simulink model "LKAS"  (R2018a)
settings: Solver=VariableStepAuto  StartTime=0.0  StopTime=50  RelTol=1e-3
undefined symbols (not defined in the file): gray, Rec, SDTV
libraries: visiongeotforms x4, visionsinks x4, vrlib x4, visionconversions x2, visiontextngfix x2, simulink x1, dspvision x1
settings Model: Creator=Aral_Sarrafi  LastModifiedBy=Aral_Sarrafi

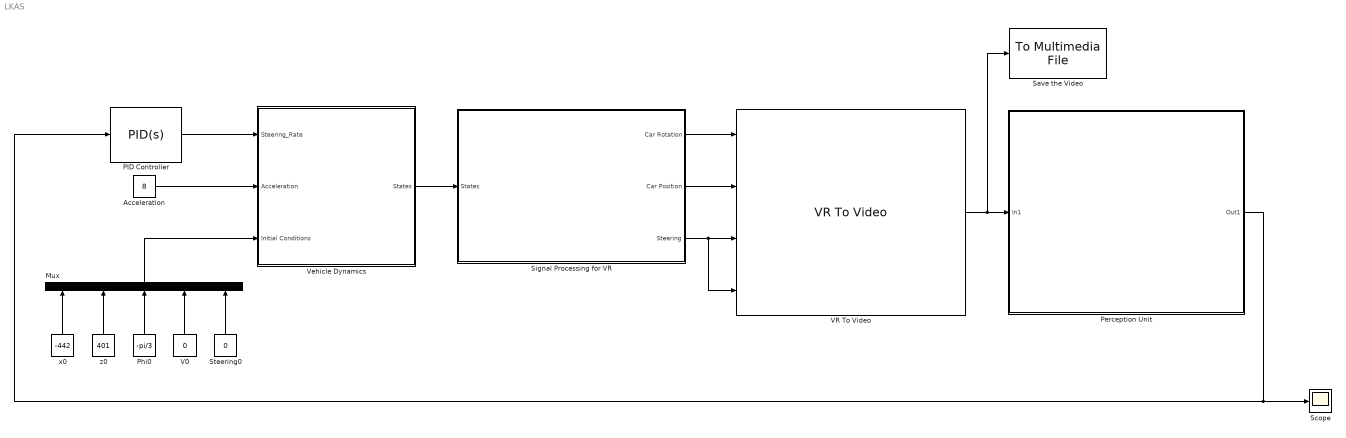
== system LKAS ==
  Acceleration : Constant  Value=8
  Mux : Mux  Inputs=5
  PID Controller : simulink/Continuous/PID Controller  Controller=PID  TimeDomain=Continuous-time  SampleTime=-1  IntegratorMethod=Forward Euler  FilterMethod=Forward Euler  Form=Parallel  UseFilter=on  ControllerParametersSource=internal  P=0.015  I=0.02  D=0.012  N=100  InitialConditionSource=internal  InitialConditionForIntegrator=0  InitialConditionForFilter=0  ExternalReset=none  LimitOutput=on  UpperSaturationLimit=pi/2  LowerSaturationLimit=-pi/2  LinearizeAsGain=off  AntiWindupMode=back-calculation  Kb=1  TrackingMode=off  Kt=1  PParamMin=[]  PParamMax=[]  IParamMin=[]  IParamMax=[]  DParamMin=[]  DParamMax=[]  NParamMin=[]  NParamMax=[]  KbParamMin=[]  KbParamMax=[]  KtParamMin=[]  KtParamMax=[]  POutMin=[]  POutMax=[]  IOutMin=[]  IOutMax=[]  DOutMin=[]  DOutMax=[]  NOutMin=[]  NOutMax=[]  KbOutMin=[]  KbOutMax=[]  KtOutMin=[]  KtOutMax=[]  IntegratorOutMin=[]  IntegratorOutMax=[]  FilterOutMin=[]  FilterOutMax=[]  SumOutMin=[]  SumOutMax=[]  SumI1OutMin=[]  SumI1OutMax=[]  SumI2OutMin=[]  SumI2OutMax=[]  SumI3OutMin=[]  SumI3OutMax=[]  SumDOutMin=[]  SumDOutMax=[]  SaturationOutMin=[]  SaturationOutMax=[]  IntegratorContinuousStateAttributes=''  IntegratorStateMustResolveToSignalObject=off  IntegratorRTWStateStorageClass=Auto  FilterContinuousStateAttributes=''  FilterStateMustResolveToSignalObject=off  FilterRTWStateStorageClass=Auto  DifferentiatorICPrevScaledInput=0  DifferentiatorOutMin=[]  DifferentiatorOutMax=[]  FilterDiffOutCoefMin=[]  FilterDiffOutCoefMax=[]  SumDenOutMin=[]  SumDenOutMax=[]  SumNumOutMin=[]  SumNumOutMax=[]  ReciprocalOutMin=[]  ReciprocalOutMax=[]  DivideOutMin=[]  DivideOutMax=[]  TunerSelectOption=Transfer Function Based (PID Tuner App)
  Perception Unit : Subsystem
      mask Display: image('computer-vision.jpg');
  Phi0 : Constant  Value=-pi/3
  Save the Video : dspvision/To Multimedia File  outputFilename=Final.mp4  streamSelection=Video only  videoCompressor=DV Video Encoder  audioCompressor=None (uncompressed)  imagePorts=One multidimensional signal  fileType=MPEG4  audioDatatype=Determine from input data type  fourcc=RGB  videoQuality=50  mj2000CompFactor=10
      settings: SourceProductName=Computer Vision System Toolbox  SourceProductBaseCode=VP
  Scope : Scope
  Signal Processing for VR : Subsystem
  Steering0 : Constant  Value=0
  V0 : Constant  Value=0
  VR To Video : vrlib/VR To Video  InstantiateOnLoad=on  SampleTime=0.02  ViewEnable=on  RemoteChange=off  RemoteView=off  FieldsWritten=Car.rotation.4.1.1.double#Car.translation.3.1.1.double#Front1.rotation.4.1.1.double#Front2.rotation.4.1.1.double  WorldFileName=Driving_Track.wrl  AutoView=off  VideoDimensions=[750 1200]  AllowVariableSize=off  FigureProperties="{'Position', 'Name', 'Viewpoint', 'CameraBound', 'CameraDirection', 'CameraPosition', 'CameraUpVector', 'ZoomFactor', 'Antialiasing', 'Headlight', 'Lighting', 'NavPanel', 'Sound', 'StatusBar', 'Stereo3D', 'Stereo3DCameraOffset', 'Stereo3DHIT', 'ToolBar', 'Textures', 'Transparency', 'Triad', 'Wireframe', 'NavZones', 'NavMode', 'NavSpeed', 'CaptureFileFormat', 'CaptureFileName', 'Record2DCompressMethod', 'Record2DCompressQuality', 'Record2D', 'Record2DFileName', 'Record2DFPS'; [3.0000000000000000e+01   6.0000000000000000e+01   1.2000000000000000e+03   7.5000000000000000e+02], '', '_untitled_1', 'on', [0.0000000000000000e+00   0.0000000000000000e+00  -1.0000000000000000e+00], [0.0000000000000000e+00   0.0000000000000000e+00   0.0000000000000000e+00], [0.0000000000000000e+00   1.0000000000000000e+00   0.0000000000000000e+00], [1.0000000000000000e+00], 'on', 'on', 'on', 'none', 'on', 'off', 'off', [1.0000000149011612e-01], [0.0000000000000000e+00], 'off', 'on', 'on', 'none', 'off', 'off', 'fly', 'normal', 'tif', '%f_anim_%n.tif', 'auto', [7.5000000000000000e+01], 'off', '***video***', 'auto'}"
      settings: SourceProductName=Simulink 3D Animation  SourceProductBaseCode=VR
  Vehicle Dynamics : Subsystem
  x0 : Constant  Value=-442
  z0 : Constant  Value=401
  wires:
  VR To Video/1 -> Save the Video/1, Perception Unit/1(In1)
  Perception Unit/1(Out1) -> PID Controller/1, Scope/1
  Signal Processing for VR/1(Car Rotation) -> VR To Video/1
  Signal Processing for VR/2(Car Position) -> VR To Video/2
  Signal Processing for VR/3(Steering) -> VR To Video/4, VR To Video/3
  PID Controller/1 -> Vehicle Dynamics/1(Steering_Rate)
  Vehicle Dynamics/1(States) -> Signal Processing for VR/1(States)
  Acceleration/1 -> Vehicle Dynamics/2(Acceleration)
  V0/1 -> Mux/4
  Phi0/1 -> Mux/3
  z0/1 -> Mux/2
  x0/1 -> Mux/1
  Mux/1 -> Vehicle Dynamics/3(Initial Conditions)
  Steering0/1 -> Mux/5

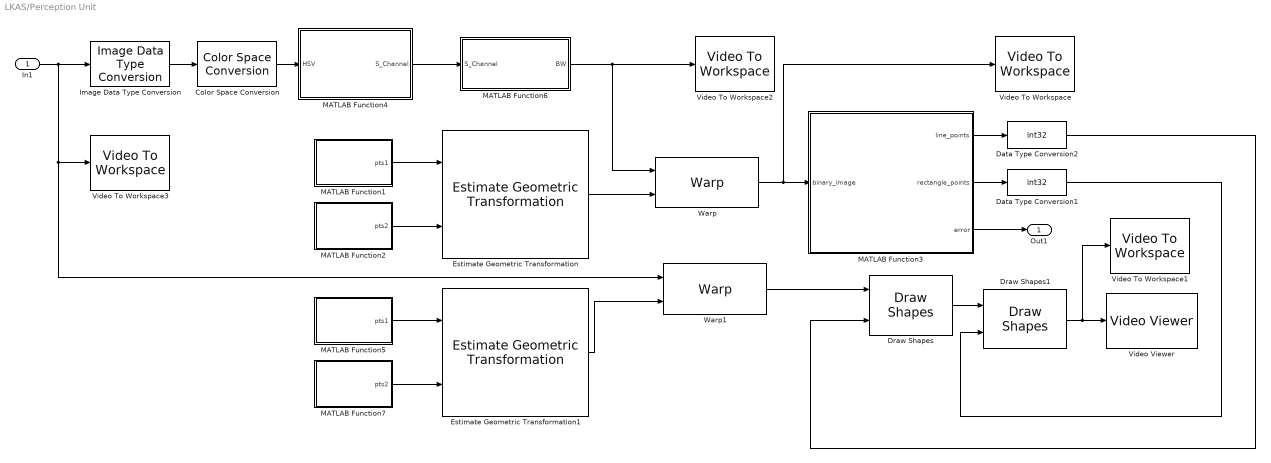
== system LKAS/Perception Unit ==
  In1 : Inport
  Color Space Conversion : visionconversions/Color Space  Conversion  conversion=Obsolete  conversionActive=R'G'B' to HSV  wp_str=D65  rec=Rec. 601 (SDTV)  sys=1125/60/2:1  imagePorts=One multidimensional signal
      settings: SourceProductName=Computer Vision System Toolbox
  Data Type Conversion1 : DataTypeConversion  OutDataTypeStr=int32
  Data Type Conversion2 : DataTypeConversion  OutDataTypeStr=int32
  Draw Shapes : visiontextngfix/Draw Shapes  shape=Lines  fill=off  lineWidth=4  fillClrSource=Specify via dialog  display=User-specified value  intensity=200  color=[255 0 0]  opacity=0.6  viewport=Entire image  antialiasing=off  inType=Obsolete  imagePorts=One multidimensional signal  prodOutputMode=Binary point scaling  prodOutputWordLength=32  prodOutputFracLength=14  memoryMode=Specify word length  memoryWordLength=16  memoryFracLength=14  roundingMode=Floor  overflowMode=off
      settings: SourceProductName=Computer Vision System Toolbox
  Draw Shapes1 : visiontextngfix/Draw Shapes  shape=Rectangles  fill=off  lineWidth=1  fillClrSource=Specify via dialog  display=User-specified value  intensity=200  color=[0 255 0]  opacity=0.6  viewport=Entire image  antialiasing=off  inType=Obsolete  imagePorts=One multidimensional signal  prodOutputMode=Binary point scaling  prodOutputWordLength=32  prodOutputFracLength=14  memoryMode=Specify word length  memoryWordLength=16  memoryFracLength=15  roundingMode=Floor  overflowMode=off
      settings: SourceProductName=Computer Vision System Toolbox
  Estimate Geometric Transformation : visiongeotforms/Estimate Geometric Transformation  tformType=Projective  isRandomSampling=on  algMethod=Random Sample Consensus (RANSAC)  distanceAlg=2.5  distanceGeo=2.5  numMethod=Specified value  sampleNum=500  desiredConfidence=99  maxSampleNum=1000  isStopSampling=off  percentStop=75  isRefineTForm=off  isReleaseMode=on  isOutputInlier=off  outDT4IntInput=Obsolete10a  outDT4IntInputActive=Single  isVarSizeAllowed=on
      settings: SourceProductName=Computer Vision System Toolbox  SourceProductBaseCode=VP
  Estimate Geometric Transformation1 : visiongeotforms/Estimate Geometric Transformation  tformType=Projective  isRandomSampling=on  algMethod=Random Sample Consensus (RANSAC)  distanceAlg=2.5  distanceGeo=2.5  numMethod=Specified value  sampleNum=500  desiredConfidence=99  maxSampleNum=1000  isStopSampling=off  percentStop=75  isRefineTForm=off  isReleaseMode=on  isOutputInlier=off  outDT4IntInput=Obsolete10a  outDT4IntInputActive=Single  isVarSizeAllowed=on
      settings: SourceProductName=Computer Vision System Toolbox  SourceProductBaseCode=VP
  Image Data Type Conversion : visionconversions/Image Data Type Conversion  outDT=double  isSigned=on  wordLen=16  numFracBits=0
      settings: SourceProductName=Computer Vision System Toolbox  SourceProductBaseCode=VP
  MATLAB Function1 : MATLAB Function  TreatAsAtomicUnit=on
  MATLAB Function2 : MATLAB Function  TreatAsAtomicUnit=on
  MATLAB Function3 : MATLAB Function  TreatAsAtomicUnit=on
  MATLAB Function4 : MATLAB Function  TreatAsAtomicUnit=on
  MATLAB Function5 : MATLAB Function  TreatAsAtomicUnit=on
  MATLAB Function6 : MATLAB Function  TreatAsAtomicUnit=on
  MATLAB Function7 : MATLAB Function  TreatAsAtomicUnit=on
  Video To Workspace : visionsinks/Video To Workspace  VariableName=warped  NumInputs=1  DataLimit=251  DecimationFactor=2  LogFi=off  InPortLabels=R|G|B
      settings: SourceProductName=Computer Vision System Toolbox  SourceProductBaseCode=VP
  Video To Workspace1 : visionsinks/Video To Workspace  VariableName=Detection  NumInputs=1  DataLimit=251  DecimationFactor=2  LogFi=off  InPortLabels=R|G|B
      settings: SourceProductName=Computer Vision System Toolbox  SourceProductBaseCode=VP
  Video To Workspace2 : visionsinks/Video To Workspace  VariableName=BW  NumInputs=1  DataLimit=500  DecimationFactor=1  LogFi=off  InPortLabels=R|G|B
      settings: SourceProductName=Computer Vision System Toolbox  SourceProductBaseCode=VP
  Video To Workspace3 : visionsinks/Video To Workspace  VariableName=Camera  NumInputs=1  DataLimit=500  DecimationFactor=1  LogFi=off  InPortLabels=R|G|B
      settings: SourceProductName=Computer Vision System Toolbox  SourceProductBaseCode=VP
  Video Viewer : VideoViewer  colormapValue=gray(256)  FigPos=[-1919 1038 1920 938]
  Warp : visiongeotforms/Warp  TransformMatrixSource=Input port  TransformMatrix=eye( 3 )  InterpolationMethod=Bilinear  BackgroundFillValue=0  OutputImagePositionSource=Same as input image  OutputImagePosition=[ 1, 1, 512, 512 ]  ROIInputPort=off  ROIValidityOutputPort=off  SimulateUsing=Interpreted execution
      settings: SourceProductName=Computer Vision System Toolbox  SourceProductBaseCode=VP
  Warp1 : visiongeotforms/Warp  TransformMatrixSource=Input port  TransformMatrix=eye( 3 )  InterpolationMethod=Bilinear  BackgroundFillValue=0  OutputImagePositionSource=Same as input image  OutputImagePosition=[ 1, 1, 512, 512 ]  ROIInputPort=off  ROIValidityOutputPort=off  SimulateUsing=Interpreted execution
      settings: SourceProductName=Computer Vision System Toolbox  SourceProductBaseCode=VP
  Out1 : Outport
  wires:
  MATLAB Function1/1(pts1) -> Estimate Geometric Transformation/1
  Estimate Geometric Transformation/1 -> Warp/2
  MATLAB Function2/1(pts2) -> Estimate Geometric Transformation/2
  MATLAB Function3/3(error) -> Out1/1
  Color Space Conversion/1 -> MATLAB Function4/1(HSV)
  Warp1/1 -> Draw Shapes/1
  Data Type Conversion2/1 -> Draw Shapes/2
  MATLAB Function7/1(pts2) -> Estimate Geometric Transformation1/2
  MATLAB Function5/1(pts1) -> Estimate Geometric Transformation1/1
  In1/1 -> Warp1/1, Video To Workspace3/1, Image Data Type Conversion/1
  Estimate Geometric Transformation1/1 -> Warp1/2
  Image Data Type Conversion/1 -> Color Space Conversion/1
  Draw Shapes/1 -> Draw Shapes1/1
  MATLAB Function3/2(rectangle_points) -> Data Type Conversion1/1
  MATLAB Function3/1(line_points) -> Data Type Conversion2/1
  Data Type Conversion1/1 -> Draw Shapes1/2
  Draw Shapes1/1 -> Video To Workspace1/1, Video Viewer/1
  MATLAB Function6/1(BW) -> Video To Workspace2/1, Warp/1
  MATLAB Function4/1(S_Channel) -> MATLAB Function6/1(S_Channel)
  Warp/1 -> Video To Workspace/1, MATLAB Function3/1(binary_image)

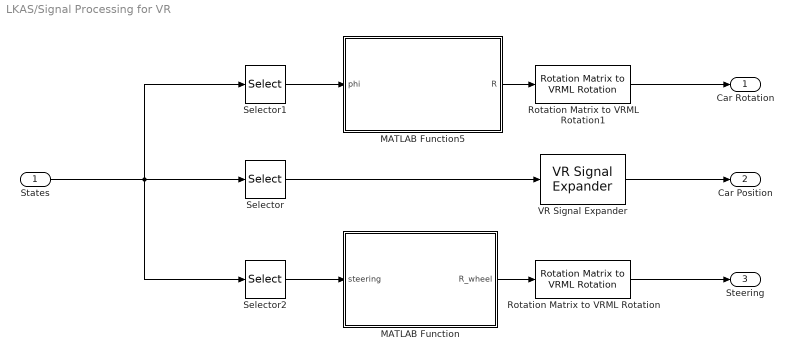
== system LKAS/Signal Processing for VR ==
  States : Inport
  MATLAB Function : MATLAB Function  TreatAsAtomicUnit=on
  MATLAB Function5 : MATLAB Function  TreatAsAtomicUnit=on
  Rotation Matrix to VRML Rotation : vrlib/Utilities/Rotation Matrix to VRML Rotation  maxzero=1e-12
      settings: SourceProductName=Simulink 3D Animation  SourceProductBaseCode=VR
  Rotation Matrix to VRML Rotation1 : vrlib/Utilities/Rotation Matrix to VRML Rotation  maxzero=1e-12
      settings: SourceProductName=Simulink 3D Animation  SourceProductBaseCode=VR
  Selector : Selector  InputPortWidth=5  IndexOptions=Index vector (dialog)  Indices=[1 2]  OutputSizes=1
  Selector1 : Selector  InputPortWidth=5  IndexOptions=Index vector (dialog)  Indices=[3]  OutputSizes=1
  Selector2 : Selector  InputPortWidth=5  IndexOptions=Index vector (dialog)  Indices=[5]  OutputSizes=1
  VR Signal Expander : vrlib/VR Signal Expander  outwidth=3  outidx=[1 3]
      settings: SourceProductName=Simulink 3D Animation  SourceProductBaseCode=VR
  Car Rotation : Outport
  Car Position : Outport  Port=2
  Steering : Outport  Port=3
  wires:
  MATLAB Function5/1(R) -> Rotation Matrix to VRML Rotation1/1
  Selector1/1 -> MATLAB Function5/1(phi)
  Selector/1 -> VR Signal Expander/1
  VR Signal Expander/1 -> Car Position/1
  MATLAB Function/1(R_wheel) -> Rotation Matrix to VRML Rotation/1
  Rotation Matrix to VRML Rotation1/1 -> Car Rotation/1
  Selector2/1 -> MATLAB Function/1(steering)
  Rotation Matrix to VRML Rotation/1 -> Steering/1
  States/1 -> Selector2/1, Selector1/1, Selector/1

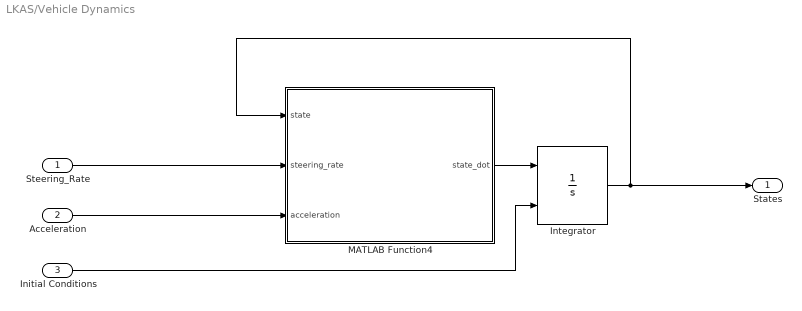
== system LKAS/Vehicle Dynamics ==
  Steering_Rate : Inport
  Acceleration : Inport  Port=2
  Initial Conditions : Inport  Port=3
  Integrator : Integrator  InitialConditionSource=external  InitialCondition=[392.5;0;pi/3;0;0]  LimitOutput=on  UpperSaturationLimit=[inf;inf;inf;36;pi/10]  LowerSaturationLimit=-[inf;inf;inf;0;pi/10]
  MATLAB Function4 : MATLAB Function  TreatAsAtomicUnit=on
  States : Outport
  wires:
  MATLAB Function4/1(state_dot) -> Integrator/1
  Acceleration/1 -> MATLAB Function4/3(acceleration)
  Integrator/1 -> States/1, MATLAB Function4/1(state)
  Steering_Rate/1 -> MATLAB Function4/2(steering_rate)
  Initial Conditions/1 -> Integrator/2

== matlab function LKAS/Perception Unit/MATLAB Function1 ==
  data: pts1 output
function pts1 = getpts1()

pts1 = [519 411
        675 411
        113 587
        1049 587];

end

== matlab function LKAS/Signal Processing for VR/MATLAB Function ==
  data: steering input; R_wheel output
function R_wheel = fcn(steering)

theta_x = pi/2;

R1 = [1 0 0; 0 cos(theta_x) -sin(theta_x); 0 sin(theta_x) cos(theta_x)];
steering = 2 * steering;
R2 = [cos(steering) 0 sin(steering); 0 1 0; -sin(steering) 0 cos(steering)];

R_wheel = R2 * R1;

end

== matlab function LKAS/Perception Unit/MATLAB Function2 ==
  data: pts2 output
function pts2 = getpts2()

h = 750; 
w = 1200;

pts2 = [450 0
        w-450 0
        450 h
        w-450 h];

end

== matlab function LKAS/Perception Unit/MATLAB Function3 ==
  data: line_points output; rectangle_points output; binary_image input; error output
function [line_points,rectangle_points,error]  = Lane_Detection(binary_image)

h = size(binary_image,1);
w = size(binary_image,2);

mid_h = w/2;

base = sum(binary_image(mid_h:end,:));


mid_w = w/2;

[~,locs] = findpeaks(base);
left_base = locs(1);

right_base = locs(locs - left_base > 200);
right_base = right_base(end);

nwindows = 10;

window_hight = h/nwindows;

leftx_current = left_base;
rightx_current = right_base;

margin = 80;
minpix = 40;

left_lane_index = [];
right_lane_index = [];

[nonzeroy, nonzerox] = find(binary_image);


rectangle_points = zeros(2 * nwindows,4);


for i = 0:nwindows-1
    %Loop over the windows to find the nonzero elements in the selected
    %window
        win_y_low = h - (i+1)*window_hight;
        win_y_high = h - i*window_hight;
        
        win_xleft_low = leftx_current - margin;
        win_xleft_high = leftx_current + margin;
        
        win_xright_low = rightx_current - margin;
        win_xright_high = rightx_current + margin;
        
        rectangle_points(i+1,:) = [win_xleft_low win_y_low 2*margin window_hight];
        rectangle_points(nwindows + 1 + i,:) = [win_xright_low win_y_low 2*margin window_hight];
        

        
        good_leftx_indexs = nonzerox((nonzeroy >= win_y_low) & (nonzeroy < win_y_high) & (nonzerox >= win_xleft_low) &  (nonzerox < win_xleft_high));
        good_lefty_indexs = nonzeroy((nonzeroy >= win_y_low) & (nonzeroy < win_y_high) & (nonzerox >= win_xleft_low) &  (nonzerox < win_xleft_high));
        
        good_rightx_indexs = nonzerox((nonzeroy >= win_y_low) & (nonzeroy < win_y_high) & (nonzerox >= win_xright_low) &  (nonzerox < win_xright_high));
        good_righty_indexs = nonzeroy((nonzeroy >= win_y_low) & (nonzeroy < win_y_high) & (nonzerox >= win_xright_low) &  (nonzerox < win_xright_high));
        
        left_lane_index = [left_lane_index; [good_leftx_indexs good_lefty_indexs]];
        right_lane_index = [right_lane_index; [good_rightx_indexs good_righty_indexs]];
        
        if(numel(good_leftx_indexs) > minpix)
            leftx_current = mean(good_leftx_indexs);
            
        end
        
        if(numel(good_rightx_indexs) > minpix)
            rightx_current = mean(good_rightx_indexs);
            
        end
          
end


p_left = polyfit(left_lane_index(:,2),left_lane_index(:,1),2);
p_right = polyfit(right_lane_index(:,2),right_lane_index(:,1),2);

y = 0:1:h;

xleft = polyval(p_left,y);
xright = polyval(p_right,y);

left_points = [xleft; y];
left_points = left_points(:)';

right_points = [xright; y];
right_points = right_points(:)';


line_points = [left_points;right_points];
error = mid_w - (xleft(end)+xright(end))/2;


end

== matlab function LKAS/Vehicle Dynamics/MATLAB Function4 ==
  data: state input; state_dot output; steering_rate input; acceleration input
function state_dot = Vehicle_Dynamics(state,steering_rate, acceleration)

    L = 4;
    %state = [x;z;si;v,steering_rate];

    phi = state(3);
    v = state(4);
    steering = state(5);

    x_dot = -v * cos (phi + steering);
    z_dot = v * sin (phi + steering);
    phi_dot = (v/L) * sin(steering);
    v_dot = acceleration;
    steering_dot = steering_rate;

    state_dot = [x_dot;z_dot;phi_dot;v_dot;steering_dot];
    

end

== matlab function LKAS/Signal Processing for VR/MATLAB Function5 ==
  data: phi input; R output
function R = fcn(phi)

R = [cos(phi) 0 sin(phi); 0 1 0; -sin(phi) 0 cos(phi)];

end

== matlab function LKAS/Perception Unit/MATLAB Function6 ==
  data: BW output; S_Channel input
function BW = mask(S_Channel)
S_th = 0.75;

BW = S_Channel > S_th;

end

== matlab function LKAS/Perception Unit/MATLAB Function4 ==
  data: S_Channel output; HSV input
function S_Channel = get_SChannel(HSV)

S_Channel = HSV(:,:,2);

end

== matlab function LKAS/Perception Unit/MATLAB Function5 ==
  data: pts1 output
function pts1 = getpts1()

pts1 = [519 411
        675 411
        113 587
        1049 587];

end

== matlab function LKAS/Perception Unit/MATLAB Function7 ==
  data: pts2 output
function pts2 = getpts2()

h = 750; 
w = 1200;

pts2 = [450 0
        w-450 0
        450 h
        w-450 h];

end
